simulink library "Wall_with_Window"  (R2013b)
settings: Solver=ode45  StartTime=0.0  StopTime=10.0  RelTol=1e-3
libraries: carnot x2
settings Model: Creator=lena.frank  LastModifiedBy=drhf

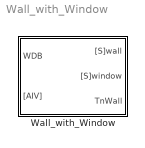
== system Wall_with_Window ==
  Wall_with_Window : Subsystem  mask(outer wall with window){wallsize=[2.5 5], windowsize=[1 2], frame=0.1, pos=0, t0=20, tau=1000*3600, g=0.7}
      mask prompts: wallsize "size of wall[m] [height width]"; windowsize "size of window[m] [height width]"; frame "part of frame of the window-surface (0..1)"; pos "azimut of wall (0=south, east= -90)]"; t0 "initial temperature [degree centigrade]"; tau "time-constant of wall and window [s]"; g "energy transmission of window"
      mask help:
      | This is the model of an outer wall with window.
      | first element of the vector = layer to surrounding
      | last element of the vector = layer to room
      mask init:
      | pos = [90 pos 0]; % position is [inclination azimut rotation]
      mask Help: web(fullfile(path_carnot('help'),'Wall_with_Window.html'),'-helpbrowser')

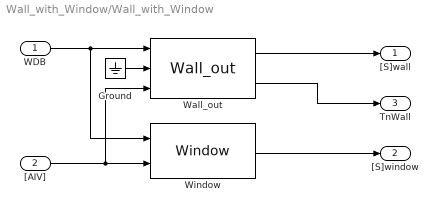
== system Wall_with_Window/Wall_with_Window ==
  WDB : Inport
  "[AIV]" : Inport  Port=2
  Ground : Ground
  Wall_out : carnot/Load/Houses/wall_floor/Wall_out  wallsize=[wallsize(1), wallsize(2)-windowsize(1)*windowsize(2)/wallsize(1)]  pos=pos  t0=t0  d=[0.1 0.38]  cond=[0.04 0.79]  cwall=[0.28 0.28]*3600  rho=[900 1800]  reflectground=0.3  abs_emiss=[0.65 0.97 0.96]  tau=tau  dactive=-1
  Window : carnot/Load/Houses/wall_floor/Window  windowsize=windowsize  frame=frame  pos=pos  t0=t0  d=[0.03 0.03]  cond=[.81 .81]  cwall=[.28 .28]*3600  rho=[2500 2500]  misc=[0.2 0.1 1 1]  gvalue=g  tau=tau  dactive=[0.01 0.05]
  "[S]wall" : Outport
  "[S]window" : Outport  Port=2
  TnWall : Outport  Port=3
  wires:
  Wall_out/2 -> TnWall/1
  WDB/1 -> Wall_out/1, Window/1
  "[AIV]"/1 -> Wall_out/3, Window/2
  Ground/1 -> Wall_out/2
  Wall_out/1 -> "[S]wall"/1
  Window/1 -> "[S]window"/1
